simulink library "MTB"  (R2014b)
settings: Solver=ode45  StartTime=0.0  StopTime=10.0  RelTol=1e-3
undefined symbols (not defined in the file or in its folder): ConfParam
libraries: ChangeFrame x1, CrossProd x1
settings Model: Creator=Hp  LastModifiedBy=Hp

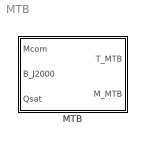
== system MTB ==
  MTB : Subsystem

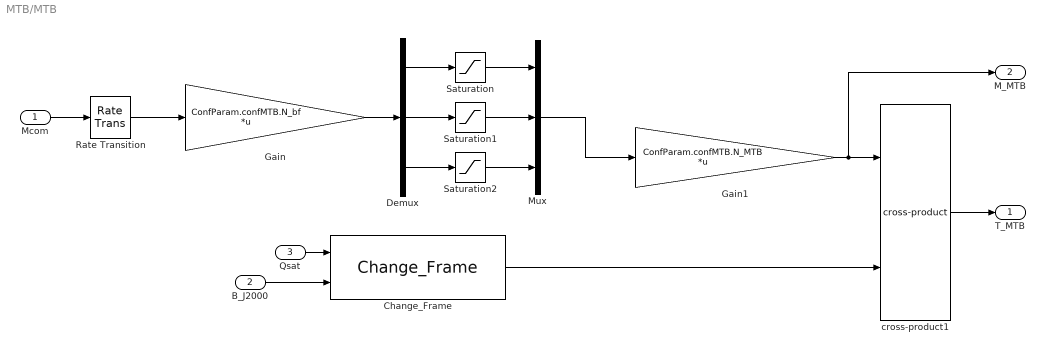
== system MTB/MTB ==
  Mcom : Inport
  B_J2000 : Inport  Port=2
  Qsat : Inport  Port=3
  Change_Frame : ChangeFrame/Change_Frame
  Demux : Demux  Outputs=3
  Gain : Gain  Gain=ConfParam.confMTB.N_bf  Multiplication=Matrix(K*u)
  Gain1 : Gain  Gain=ConfParam.confMTB.N_MTB  Multiplication=Matrix(K*u)
  Mux : Mux  Inputs=3
  Rate Transition : RateTransition  X0=[0;0;0]  OutPortSampleTime=ConfParam.confOrbit.dt
  Saturation : Saturate  UpperLimit=ConfParam.confMTB.M_max  LowerLimit=-ConfParam.confMTB.M_max
  Saturation1 : Saturate  UpperLimit=ConfParam.confMTB.M_max  LowerLimit=-ConfParam.confMTB.M_max
  Saturation2 : Saturate  UpperLimit=ConfParam.confMTB.M_max  LowerLimit=-ConfParam.confMTB.M_max
  cross-product1 : CrossProd/cross-product
  T_MTB : Outport
  M_MTB : Outport  Port=2
  wires:
  Demux/1 -> Saturation/1
  Demux/3 -> Saturation2/1
  Demux/2 -> Saturation1/1
  Saturation/1 -> Mux/1
  Saturation1/1 -> Mux/2
  Saturation2/1 -> Mux/3
  Mux/1 -> Gain1/1
  B_J2000/1 -> Change_Frame/2
  cross-product1/1 -> T_MTB/1
  Gain1/1 -> cross-product1/1, M_MTB/1
  Mcom/1 -> Rate Transition/1
  Gain/1 -> Demux/1
  Qsat/1 -> Change_Frame/1
  Change_Frame/1 -> cross-product1/2
  Rate Transition/1 -> Gain/1
